simulink model "test_distributed_parameter_line"  (R2025b)
settings: Solver=FixedStepAuto  StartTime=0.0  StopTime=2  RelTol=1e-3
PreLoadFcn:
  | length = 100;
  | 
  | R3m = [0.10710 0.09729 0.09499
  |        0.09729 0.11050 0.09729
  |        0.09499 0.09729 0.10710];
  | 
  | L3m = [0.00158 0.00075 0.00062
  |        0.00075 0.00157 0.00075
  |        0.00062 0.00075 0.00158];
  | 
  | C3m = [1.16613e-8  -2.12683e-9 -5.83623e-10
  |       -2.12683e-9   1.21174e-8 -2.12683e-9
  |       -5.83623e-10 -2.12683e-9  1.16613e-8];
  | 
  | 
  | Ts = 5e-5;
libraries: ee_lib x8, nesl_utility x6, fl_lib x1
settings Model: Creator=gdudgeon  LastModifiedBy=gdudgeon

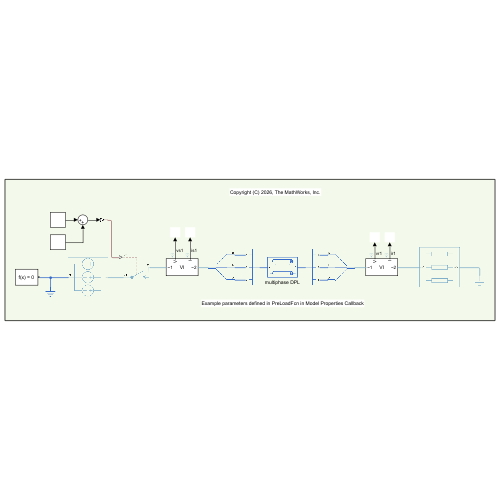
[thumbnail: Simulink's stored preview of the top-level diagram]
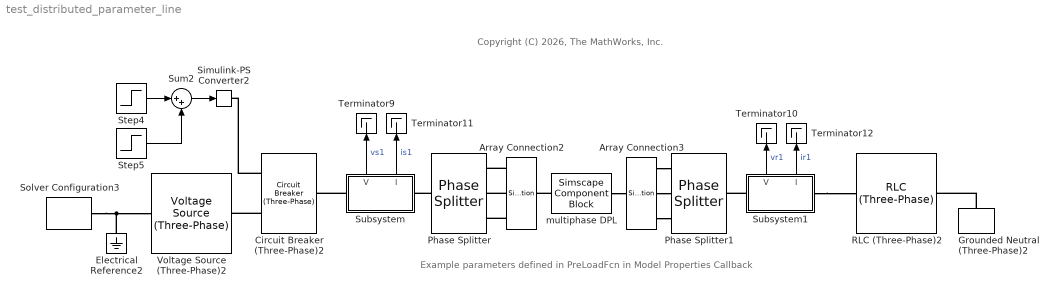
== system test_distributed_parameter_line ==
  note: Example parameters defined in PreLoadFcn in Model Properties Callback
  note: Copyright (C) 2026, The MathWorks, Inc.
  Array Connection2 : SimscapeArrayConnection  NumScalarElements=3
  Array Connection3 : SimscapeArrayConnection  NumScalarElements=3
  Circuit Breaker (Three-Phase)2 : ee_lib/Switches & Breakers/Circuit Breaker (Three-Phase)  R_closed=1e-4 Ohm  G_open=1e-6 1/Ohm  threshold=0.5 V  breaker_behavior=ee.enum.switches.breakerBehavior.zeroCrossingEnable
      settings: InternalSimscapePortConfiguration="{\"Bottom\":[],\"Left\":[{\"id\":\"vT\",\"label\":\"vT\",\"type\":\"input\"},{\"id\":\"N1\",\"label\":\"~1\",\"type\":\"foundation.electrical.three_phase\"}],\"Right\":[{\"id\":\"N2\",\"label\":\"~2\",\"type\":\"foundation.electrical.three_phase\"}],\"Top\":[]}"
  Electrical Reference2 : fl_lib/Electrical/Electrical Elements/Electrical Reference
  Grounded Neutral (Three-Phase)2 : ee_lib/Connectors & References/Grounded Neutral (Three-Phase)
  Phase Splitter : ee_lib/Connectors & References/Phase Splitter
  Phase Splitter1 : ee_lib/Connectors & References/Phase Splitter
  RLC (Three-Phase)2 : ee_lib/Passive/RLC Assemblies/RLC (Three-Phase)  port_option=ee.enum.threePhasePort.composite  component_structure=ee.enum.rlc.structure.SeriesRL  R=1 Ohm  L=1e-3 H  C=1e-6 F  R_parasitic=0 Ohm  G_parasitic=0 1/Ohm  IL_specify=off  IL_priority=High  IL=[0, 0, 0] A  IL_nominal_specify=off  IL_nominal_value=1  IL_nominal_unit=A  VC_specify=off  VC_priority=High  VC=[0, 0, 0] V  VC_nominal_specify=off  VC_nominal_value=1  VC_nominal_unit=V
      settings: InternalSimscapePortConfiguration="{\"Bottom\":[],\"Left\":[{\"id\":\"N1\",\"label\":\"~1\",\"type\":\"foundation.electrical.three_phase\"}],\"Right\":[{\"id\":\"N2\",\"label\":\"~2\",\"type\":\"foundation.electrical.three_phase\"}],\"Top\":[]}"
  Simulink-PS Converter2 : nesl_utility/Simulink-PS Converter  PhysicalDomain=network_engine_domain  SubClassName=ps_input  LeftPortType=input  RightPortType=output  PseudoPeriodic=off  Frequencies=[]  NoiseDistribution=none  NoiseParameters=[]  Unit=1  AffineConversion=off  FilteringAndDerivatives=provide  SimscapeFilterOrder=1  InputFilterTimeConstant=0.001  UdotUserProvided=0
  Solver Configuration3 : nesl_utility/Solver Configuration  PhysicalDomain=network_engine_domain  SubClassName=solver  LeftPortType=input  RightPortType=generic  Tones=[]  Harmonics=[]  SimulateNoise=off  Profile=off  UseLocalSampling=off  EnableSwitchedLinearOptims=on  FrequencyDomain=off  UseCCode=off  RelTol=0.001  AbsTol=0.001  MinStep=1e-09  ToWorkspace=off  RevertToSquareIcSolve=off  NumHomotopyIterations=100  PhasorMode=off  PhasorModeNumHarmonics=1  ConsistencySolver=NEWTON_XTOL_AFTER_FTOL  IndexReductionMethod=None  DoDC=off  ResidualTolerance=1e-09  ConsistencyTolSource=GLOBAL  ConsistencyAbsTol=0.001  ConsistencyRelTol=0.001  ConsistencyTolFactor=0.001  UseLocalSolver=on  LocalSolverChoice=NE_BACKWARD_EULER_ADVANCER  ResolveIndetEquations=off  FunctionEvalNumThread=1  LocalSolverSampleTime=Ts  DoFixedCost=on  MaxNonlinIter=1  MaxModeIter=2  ComputeImpulses=off  ImpulseIterations=2  LinearAlgebra=auto  LinearAlgebraNumThread=0  EquationFormulation=NE_TIME_EF  DelaysMemoryBudget=1024  AutomaticFiltering=off  FilteringTimeConstant=0.001  PartitionStorageMethod=AS_NEEDED  PartitionMemoryBudget=1024  PartitionMethod=ROBUST  MultibodyUseLocalSolver=off  MultibodyLocalSolverChoice=ODE1  MultibodyLocalSolverSampleTime=0.001
  Step4 : Step  SampleTime=0
  Step5 : Step  Time=1+1.3/60  After=-1  SampleTime=0
  Subsystem : Subsystem
      settings: PortSchema="{\"entries\":[{\"content\":{\"sides\":[{\"content\":{\"connectorIds\":[\"LConn1\"]},\"type\":\"ConnectorPlacement.EquallySpacedRectSide\",\"uuid\":\"c47d0818-c5fb-4b96-9f2c-43958960f24c\"},{\"content\":{\"connectorIds\":[\"RConn1\"],\"side\":\"RIGHT\"},\"type\":\"ConnectorPlacement.EquallySpacedRectSide\",\"uuid\":\"87c2ed83-26c9-4578-9de4-75c7fe05a5ee\"},{\"content\":{\"connectorIds\":[\"Out1\",\"Out2\"],\"side\":\"TOP\"},\"type\":\"ConnectorPlacement.EquallySpacedRectSide\",\"uuid\":\"b709fb5f-5815-44cd-9573-5d1fcab2fad3\"}]},\"type\":\"ConnectorPlacement.EquallySpacedConnector\",\"uuid\":\"b85a8924-d721-4ae1-a801-f3f61c80191a\"}],\"packageUris\":[\"http://schema.mathworks.com/mf0/Connector/R2020b\"],\"version\":\"1.0\"}"
      mask Display: disp('VI')
  Subsystem1 : Subsystem
      settings: PortSchema="{\"entries\":[{\"content\":{\"sides\":[{\"content\":{\"connectorIds\":[\"LConn1\"]},\"type\":\"ConnectorPlacement.EquallySpacedRectSide\",\"uuid\":\"c47d0818-c5fb-4b96-9f2c-43958960f24c\"},{\"content\":{\"connectorIds\":[\"RConn1\"],\"side\":\"RIGHT\"},\"type\":\"ConnectorPlacement.EquallySpacedRectSide\",\"uuid\":\"87c2ed83-26c9-4578-9de4-75c7fe05a5ee\"},{\"content\":{\"connectorIds\":[\"Out1\",\"Out2\"],\"side\":\"TOP\"},\"type\":\"ConnectorPlacement.EquallySpacedRectSide\",\"uuid\":\"b709fb5f-5815-44cd-9573-5d1fcab2fad3\"}]},\"type\":\"ConnectorPlacement.EquallySpacedConnector\",\"uuid\":\"b85a8924-d721-4ae1-a801-f3f61c80191a\"}],\"packageUris\":[\"http://schema.mathworks.com/mf0/Connector/R2020b\"],\"version\":\"1.0\"}"
      mask Display: disp('VI')
  Sum2 : Sum  Inputs=|++
  Terminator{9..12} (4 alike) : Terminator
  Voltage Source (Three-Phase)2 : ee_lib/Sources/Voltage Source (Three-Phase)  vline_rms=100 V  shift=0 deg  freq=60 Hz  impedance_option=0  SShortCircuit=1e6 A*V  XR=15  R=0.01 Ohm  L=3.97e-4 H  harmonic_option=0  harmonic_orders=[5, 7, 11, 13]  harmonic_ratios=[.1, .1, .1, .1]  G_parasitic=0 1/Ohm  I_specify=off  I_priority=None  I=[0, 0, 0] A  I_nominal_specify=off  I_nominal_value=1  I_nominal_unit=A
  multiphase DPL : SimscapeComponentBlock  SourceFile=mp_distributed_parameter_line  ComponentPath=mp_distributed_parameter_line  ComponentVariants="[\"mp_distributed_parameter_line\"]"  ComponentVariantNames="[\"mp_distributed_parameter_line\"]"  ClassName=mp_distributed_parameter_line  SchemaVersion=1  line_type=lineType.general  length=length km  freq=60 Hz  nPhase=3  N=1  Rs=0.02 Ohm/km  Rm=0.01 Ohm/km  Ls=0.5 mH/km  Lm=0.1 mH/km  Cs=0.7 uF/km  Cm=-0.3 uF/km  Rmat=R3m Ohm/km  Lmat=L3m*1e3 mH/km  Cmat=C3m*1e6 uF/km
      settings: CopyFcn=simscape.sscblock.internal.componentBlockCallback(gcbh,'COPY')  PreCopyFcn=simscape.sscblock.internal.componentBlockCallback(gcbh,'PRECOPY')  PreDeleteFcn=simscape.sscblock.internal.componentBlockCallback(gcbh,'PREDELETE')  InternalSimscapePortConfiguration="{\"Bottom\":[],\"Left\":[{\"id\":\"p\",\"label\":\"1\",\"type\":\"foundation.electrical.electrical\"}],\"Right\":[{\"id\":\"n\",\"label\":\"2\",\"type\":\"foundation.electrical.electrical\"}],\"Top\":[]}"
      mask Type: multiphase DPL
  wires:
  Step4/1 -> Sum2/1
  Step5/1 -> Sum2/2
  Sum2/1 -> Simulink-PS Converter2/1
  Subsystem/1(V) -> Terminator9/1  "vs1"
  Subsystem/2(I) -> Terminator11/1  "is1"
  Subsystem1/1(V) -> Terminator10/1  "vr1"
  Subsystem1/2(I) -> Terminator12/1  "ir1"
  connections:
  Solver Configuration3/RConn1 -- Electrical Reference2/LConn1 -- Voltage Source (Three-Phase)2/LConn1
  Array Connection3/LConn2 -- Phase Splitter1/RConn2
  Array Connection2/LConn3 -- Phase Splitter/RConn3
  Array Connection2/LConn1 -- Phase Splitter/RConn1
  Array Connection3/LConn1 -- Phase Splitter1/RConn1
  Circuit Breaker (Three-Phase)2/LConn2 -- Voltage Source (Three-Phase)2/RConn1
  Circuit Breaker (Three-Phase)2/LConn1 -- Simulink-PS Converter2/RConn1
  Grounded Neutral (Three-Phase)2/LConn1 -- RLC (Three-Phase)2/RConn1
  Array Connection3/LConn3 -- Phase Splitter1/RConn3
  Subsystem1/LConn1 -- Phase Splitter1/LConn1
  Array Connection2/LConn2 -- Phase Splitter/RConn2
  Subsystem1/RConn1 -- RLC (Three-Phase)2/LConn1
  Subsystem/LConn1 -- Circuit Breaker (Three-Phase)2/RConn1
  Phase Splitter/LConn1 -- Subsystem/RConn1
  multiphase DPL/RConn1 -- Array Connection2/RConn1
  multiphase DPL/LConn1 -- Array Connection3/RConn1

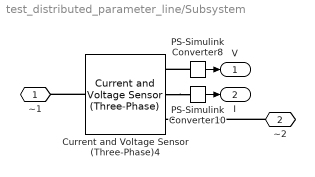
== system test_distributed_parameter_line/Subsystem ==
  Current and Voltage Sensor (Three-Phase)4 : ee_lib/Sensors & Transducers/Current and Voltage Sensor (Three-Phase)  vMeasurementType=ee.enum.vmeasurement.lg  outputUnit=ee.enum.unit.si  SRated=100e6 A*V  VRated=24e3 V  I_specify=off  I_priority=None  I=[0, 0, 0] A  I_nominal_specify=off  I_nominal_value=1  I_nominal_unit=A  V_specify=off  V_priority=None  V=[0, 0, 0] V  V_nominal_specify=off  V_nominal_value=1  V_nominal_unit=V
      settings: InternalSimscapePortConfiguration="{\"Bottom\":[],\"Left\":[{\"id\":\"N1\",\"label\":\"~1\",\"type\":\"foundation.electrical.three_phase\"}],\"Right\":[{\"id\":\"V_output\",\"label\":\"V\",\"type\":\"output\"},{\"id\":\"I_output\",\"label\":\"I\",\"type\":\"output\"},{\"id\":\"N2\",\"label\":\"~2\",\"type\":\"foundation.electrical.three_phase\"}],\"Top\":[]}"
  PS-Simulink Converter10 : nesl_utility/PS-Simulink Converter  PhysicalDomain=network_engine_domain  SubClassName=ps_output  LeftPortType=input  RightPortType=output  PseudoPeriodic=off  Frequencies=[]  VectorFormat=inherit  Unit=inherit  AffineConversion=off
  PS-Simulink Converter8 : nesl_utility/PS-Simulink Converter  PhysicalDomain=network_engine_domain  SubClassName=ps_output  LeftPortType=input  RightPortType=output  PseudoPeriodic=off  Frequencies=[]  VectorFormat=inherit  Unit=inherit  AffineConversion=off
  ~1 : PMIOPort  Side=Left
  ~2 : PMIOPort  Port=2  Side=Right
  V : Outport
  I : Outport  Port=2
  wires:
  PS-Simulink Converter10/1 -> I/1
  PS-Simulink Converter8/1 -> V/1
  connections:
  PS-Simulink Converter8/LConn1 -- Current and Voltage Sensor (Three-Phase)4/RConn1
  ~2/RConn1 -- Current and Voltage Sensor (Three-Phase)4/RConn3
  Current and Voltage Sensor (Three-Phase)4/LConn1 -- ~1/RConn1
  Current and Voltage Sensor (Three-Phase)4/RConn2 -- PS-Simulink Converter10/LConn1

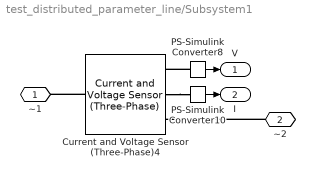
== system test_distributed_parameter_line/Subsystem1 ==
  Current and Voltage Sensor (Three-Phase)4 : ee_lib/Sensors & Transducers/Current and Voltage Sensor (Three-Phase)  vMeasurementType=ee.enum.vmeasurement.lg  outputUnit=ee.enum.unit.si  SRated=100e6 A*V  VRated=24e3 V  I_specify=off  I_priority=None  I=[0, 0, 0] A  I_nominal_specify=off  I_nominal_value=1  I_nominal_unit=A  V_specify=off  V_priority=None  V=[0, 0, 0] V  V_nominal_specify=off  V_nominal_value=1  V_nominal_unit=V
      settings: InternalSimscapePortConfiguration="{\"Bottom\":[],\"Left\":[{\"id\":\"N1\",\"label\":\"~1\",\"type\":\"foundation.electrical.three_phase\"}],\"Right\":[{\"id\":\"V_output\",\"label\":\"V\",\"type\":\"output\"},{\"id\":\"I_output\",\"label\":\"I\",\"type\":\"output\"},{\"id\":\"N2\",\"label\":\"~2\",\"type\":\"foundation.electrical.three_phase\"}],\"Top\":[]}"
  PS-Simulink Converter10 : nesl_utility/PS-Simulink Converter  PhysicalDomain=network_engine_domain  SubClassName=ps_output  LeftPortType=input  RightPortType=output  PseudoPeriodic=off  Frequencies=[]  VectorFormat=inherit  Unit=inherit  AffineConversion=off
  PS-Simulink Converter8 : nesl_utility/PS-Simulink Converter  PhysicalDomain=network_engine_domain  SubClassName=ps_output  LeftPortType=input  RightPortType=output  PseudoPeriodic=off  Frequencies=[]  VectorFormat=inherit  Unit=inherit  AffineConversion=off
  ~1 : PMIOPort  Side=Left
  ~2 : PMIOPort  Port=2  Side=Right
  V : Outport
  I : Outport  Port=2
  wires:
  PS-Simulink Converter8/1 -> V/1
  PS-Simulink Converter10/1 -> I/1
  connections:
  Current and Voltage Sensor (Three-Phase)4/RConn2 -- PS-Simulink Converter10/LConn1
  Current and Voltage Sensor (Three-Phase)4/LConn1 -- ~1/RConn1
  ~2/RConn1 -- Current and Voltage Sensor (Three-Phase)4/RConn3
  PS-Simulink Converter8/LConn1 -- Current and Voltage Sensor (Three-Phase)4/RConn1
